simulink model "IEEE30_case"  (R2024b)
settings: Solver=FixedStepAuto  StartTime=0  StopTime=5  FixedStep=1e-7  RelTol=1e-3
values from neighbouring files (symbols this model uses):
  GFL_DFIG_7_C_bus = 0.08    [IEEE30_case_parameters.m]
  GFL_DFIG_7_D_mutual = 2.500000e+3    (= 2500)    [IEEE30_case_parameters.m]
  GFL_DFIG_7_f0 = 60    [IEEE30_case_parameters.m]
  GFL_DFIG_7_gPLLi = 3200    [IEEE30_case_parameters.m]
  GFL_DFIG_7_gPLLp = 650    [IEEE30_case_parameters.m]
  GFL_DFIG_7_H_WT = 0.4    [IEEE30_case_parameters.m]
  GFL_DFIG_7_Hg = 0.8    [IEEE30_case_parameters.m]
  GFL_DFIG_7_Igq_ref = 0    [IEEE30_case_parameters.m]
  GFL_DFIG_7_Ird_ref = 704.45696    [IEEE30_case_parameters.m]
  GFL_DFIG_7_KI_V = -300000    [IEEE30_case_parameters.m]
  GFL_DFIG_7_KP_V = -1000    [IEEE30_case_parameters.m]
  GFL_DFIG_7_Ksh = 1.254300e+4    (= 12543)    [IEEE30_case_parameters.m]
  GFL_DFIG_7_Lg = 0.000483    [IEEE30_case_parameters.m]
  GFL_DFIG_7_Lm_pu = 4    [IEEE30_case_parameters.m]
  GFL_DFIG_7_N = 100    [IEEE30_case_parameters.m]
  GFL_DFIG_7_p = 2    [IEEE30_case_parameters.m]
  GFL_DFIG_7_Pitch = 0    [IEEE30_case_parameters.m]
  GFL_DFIG_7_R = 44    [IEEE30_case_parameters.m]
  GFL_DFIG_7_Rg = 2.000000e-5    (= 2e-05)    [IEEE30_case_parameters.m]
  GFL_DFIG_7_rho = 1.225    [IEEE30_case_parameters.m]
  GFL_DFIG_7_rPLLi = 4500    [IEEE30_case_parameters.m]
  GFL_DFIG_7_rPLLp = 620    [IEEE30_case_parameters.m]
  GFL_DFIG_7_Rs_pu = 0.011    [IEEE30_case_parameters.m]
  GFL_DFIG_7_Sbase = 2.000000e+6    (= 2000000)    [IEEE30_case_parameters.m]
  GFL_DFIG_7_ugq_ref = 0    [IEEE30_case_parameters.m]
  GFL_DFIG_7_usd_ref = 0    [IEEE30_case_parameters.m]
  GFL_DFIG_7_Vbase = 690    [IEEE30_case_parameters.m]
  GFL_DFIG_7_Vdc_ref = 1200    [IEEE30_case_parameters.m]
  GFL_DFIG_7_wind = 12    [IEEE30_case_parameters.m]
  GFL_DFIG_7_wm_ref = 518.184209    [IEEE30_case_parameters.m]
  SG_D_13_D = 0.01056    [IEEE30_case_parameters.m]
  SG_D_13_EnableSaturation = 0    [IEEE30_case_parameters.m]
  SG_D_13_f0 = 60    [IEEE30_case_parameters.m]
  SG_D_13_H = 7.5    [IEEE30_case_parameters.m]
  SG_D_13_K_A = 20    [IEEE30_case_parameters.m]
  SG_D_13_K_E = 1.000000e+1    (= 10)    [IEEE30_case_parameters.m]
  SG_D_13_K_F = 2.363    [IEEE30_case_parameters.m]
  SG_D_13_K_s = 0.5    [IEEE30_case_parameters.m]
  SG_D_13_R_a = 0.001088    [IEEE30_case_parameters.m]
  SG_D_13_S_A = 1    [IEEE30_case_parameters.m]
  SG_D_13_S_B = 0.103    [IEEE30_case_parameters.m]
  SG_D_13_S_N = 10.659857    [IEEE30_case_parameters.m]
  SG_D_13_SpeedPara = 200    [IEEE30_case_parameters.m]
  SG_D_13_T_0 = 0.370163    [IEEE30_case_parameters.m]
  SG_D_13_T_1 = 0.3    [IEEE30_case_parameters.m]
  SG_D_13_T_2 = 0.05    [IEEE30_case_parameters.m]
  SG_D_13_T_3 = 0.02    [IEEE30_case_parameters.m]
  SG_D_13_T_4 = 0.005    [IEEE30_case_parameters.m]
  SG_D_13_T_A = 0.02    [IEEE30_case_parameters.m]
  SG_D_13_T_dd = 8.000000e+0    (= 8)    [IEEE30_case_parameters.m]
  SG_D_13_T_ddd = 0.04    [IEEE30_case_parameters.m]
  SG_D_13_T_E = 0.314    [IEEE30_case_parameters.m]
  SG_D_13_T_F = 0.35    [IEEE30_case_parameters.m]
  SG_D_13_T_qd = 0.8    [IEEE30_case_parameters.m]
  SG_D_13_T_qdd = 0.02    [IEEE30_case_parameters.m]
  SG_D_13_T_speed = 0.1    [IEEE30_case_parameters.m]
  SG_D_13_T_w = 0.5    [IEEE30_case_parameters.m]
  SG_D_13_V_ref = 1.696619    [IEEE30_case_parameters.m]
  SG_D_13_w_ref = 376.991118    [IEEE30_case_parameters.m]
  SG_D_13_x_d = 1.9    [IEEE30_case_parameters.m]
  SG_D_13_x_dd = 0.302    [IEEE30_case_parameters.m]
  SG_D_13_x_ddd = 0.204    [IEEE30_case_parameters.m]
  SG_D_13_x_l = 0.05    [IEEE30_case_parameters.m]
  SG_D_13_x_q = 1.3    [IEEE30_case_parameters.m]
  SG_D_13_x_qd = 0.5    [IEEE30_case_parameters.m]
  SG_D_13_x_qdd = 0.3    [IEEE30_case_parameters.m]
  SG_D_1_D = 0.01056    [IEEE30_case_parameters.m]
  SG_D_1_EnableSaturation = 0    [IEEE30_case_parameters.m]
  SG_D_1_f0 = 60    [IEEE30_case_parameters.m]
  SG_D_1_H = 7.5    [IEEE30_case_parameters.m]
  SG_D_1_K_A = 20    [IEEE30_case_parameters.m]
  SG_D_1_K_E = 1.000000e+1    (= 10)    [IEEE30_case_parameters.m]
  SG_D_1_K_F = 2.363    [IEEE30_case_parameters.m]
  SG_D_1_K_s = 0.5    [IEEE30_case_parameters.m]
  SG_D_1_R_a = 0.001088    [IEEE30_case_parameters.m]
  SG_D_1_S_A = 1    [IEEE30_case_parameters.m]
  SG_D_1_S_B = 0.103    [IEEE30_case_parameters.m]
  SG_D_1_S_N = 10.659857    [IEEE30_case_parameters.m]
  SG_D_1_SpeedPara = 200    [IEEE30_case_parameters.m]
  SG_D_1_T_0 = 0.259812    [IEEE30_case_parameters.m]
  SG_D_1_T_1 = 0.3    [IEEE30_case_parameters.m]
  SG_D_1_T_2 = 0.05    [IEEE30_case_parameters.m]
  SG_D_1_T_3 = 0.02    [IEEE30_case_parameters.m]
  SG_D_1_T_4 = 0.005    [IEEE30_case_parameters.m]
  SG_D_1_T_A = 0.02    [IEEE30_case_parameters.m]
  SG_D_1_T_dd = 8.000000e+0    (= 8)    [IEEE30_case_parameters.m]
  SG_D_1_T_ddd = 0.04    [IEEE30_case_parameters.m]
  SG_D_1_T_E = 0.314    [IEEE30_case_parameters.m]
  SG_D_1_T_F = 0.35    [IEEE30_case_parameters.m]
  SG_D_1_T_qd = 0.8    [IEEE30_case_parameters.m]
  SG_D_1_T_qdd = 0.02    [IEEE30_case_parameters.m]
  SG_D_1_T_speed = 0.1    [IEEE30_case_parameters.m]
  SG_D_1_T_w = 0.5    [IEEE30_case_parameters.m]
  SG_D_1_V_ref = 1.544107    [IEEE30_case_parameters.m]
  SG_D_1_w_ref = 376.991118    [IEEE30_case_parameters.m]
  SG_D_1_x_d = 1.9    [IEEE30_case_parameters.m]
  SG_D_1_x_dd = 0.302    [IEEE30_case_parameters.m]
  SG_D_1_x_ddd = 0.204    [IEEE30_case_parameters.m]
  SG_D_1_x_l = 0.05    [IEEE30_case_parameters.m]
  SG_D_1_x_q = 1.3    [IEEE30_case_parameters.m]
  SG_D_1_x_qd = 0.5    [IEEE30_case_parameters.m]
  SG_D_1_x_qdd = 0.3    [IEEE30_case_parameters.m]
  SG_D_22_D = 0.01056    [IEEE30_case_parameters.m]
  SG_D_22_EnableSaturation = 0    [IEEE30_case_parameters.m]
  SG_D_22_f0 = 60    [IEEE30_case_parameters.m]
  SG_D_22_H = 7.5    [IEEE30_case_parameters.m]
  SG_D_22_K_A = 20    [IEEE30_case_parameters.m]
  SG_D_22_K_E = 1.000000e+1    (= 10)    [IEEE30_case_parameters.m]
  SG_D_22_K_F = 2.363    [IEEE30_case_parameters.m]
  SG_D_22_K_s = 0.5    [IEEE30_case_parameters.m]
  SG_D_22_R_a = 0.001088    [IEEE30_case_parameters.m]
  SG_D_22_S_A = 1    [IEEE30_case_parameters.m]
  SG_D_22_S_B = 0.103    [IEEE30_case_parameters.m]
  SG_D_22_S_N = 10.659857    [IEEE30_case_parameters.m]
  SG_D_22_SpeedPara = 200    [IEEE30_case_parameters.m]
  SG_D_22_T_0 = 0.216121    [IEEE30_case_parameters.m]
  SG_D_22_T_1 = 0.3    [IEEE30_case_parameters.m]
  SG_D_22_T_2 = 0.05    [IEEE30_case_parameters.m]
  SG_D_22_T_3 = 0.02    [IEEE30_case_parameters.m]
  SG_D_22_T_4 = 0.005    [IEEE30_case_parameters.m]
  ... (+126 more)
(part 23 of 27)

== system IEEE30_case/SG_D_22/d_w_SG_D_22_block ==
  note: d_w_SG_D_22 in IEEE30_case
      | $\frac{2\,\pi \,T_{m,\mathrm{SG},D,22}\,f_{0}-D\,\left(w_{\mathrm{SG},D,22}-2\,\pi \,f_{0}\right)+2\,\pi \,f_{0}\,\left(\frac{\psi _{d,\mathrm{SG},D,22}\,\left(\psi _{q,\mathrm{SG},D,22}+\frac{\psi _{\mathrm{gq},\mathrm{SG},D,22}\,\left(x_{l}-x_{\mathrm{qdd}}\right)}{x_{l}-x_{\mathrm{qd}}}+\frac{\psi _{\mathrm{kq},\mathrm{SG},D,22}\,\left(x_{\mathrm{qd}}-x_{\mathrm{qdd}}\right)}{x_{l}-x_{\mathrm{qd}}}\right)}{x_{\mathrm{qdd}}}+\frac{\psi _{q,\mathrm{SG},D,22}\,\left(\frac{\psi _{\mathrm{1d},\mathrm{SG},D,22}\,\left(x_{\mathrm{dd}}-x_{\mathrm{ddd}}\right)}{x_{\mathrm{dd}}-x_{l}}-\psi _{d,\mathrm{SG},D,22}+\frac{\psi _{\mathrm{fd},\mathrm{SG},D,22}\,\left(x_{\mathrm{ddd}}-x_{l}\right)}{x_{\mathrm{dd}}-x_{l}}\right)}{x_{\mathrm{ddd}}}\right)}{2\,H}$
      | Automatically generated on 2025-11-01 18:36:16 .
  State_w_SG_D_22_fa999 : Inport
  State_T_m_SG_D_22_7e244 : Inport  Port=2
  State_psi_d_SG_D_22_73560 : Inport  Port=3
  State_psi_gq_SG_D_22_bb4d3 : Inport  Port=4
  State_psi_kq_SG_D_22_23ee7 : Inport  Port=5
  State_psi_q_SG_D_22_4ef4a : Inport  Port=6
  State_psi_q_SG_D_22_8c90d : Inport  Port=7
  State_psi_1d_SG_D_22_62d4d : Inport  Port=8
  State_psi_d_SG_D_22_0b647 : Inport  Port=9
  State_psi_fd_SG_D_22_b8daa : Inport  Port=10
  Add_01781 : Sum
  Add_114db : Sum
  Add_20ea4 : Sum
  Add_483be : Sum
  Add_4e463 : Sum
  Add_6d455 : Sum
  Add_81a44 : Sum
  Add_86346 : Sum
  Constant_-1_0835d : Constant  Value=-1
  Constant_-1_479f7 : Constant  Value=-1
  Constant_-1_4ac95 : Constant  Value=-1
  Constant_-1_7f41a : Constant  Value=-1
  Constant_-1_aceb8 : Constant  Value=-1
  Constant_-1_ccaa9 : Constant  Value=-1
  Constant_-2.0_91187 : Constant  Value=-2.0
  Constant_2.0_035fa : Constant  Value=2.0
  Constant_2.0_a509c : Constant  Value=2.0
  Constant_2.0_ee757 : Constant  Value=2.0
  Constant_D_fe311 : Constant  Value=D
  Constant_H_e5a3f : Constant  Value=H
  Constant_f0_a860d : Constant  Value=f0
  Constant_f0_ea105 : Constant  Value=f0
  Constant_f0_f8cec : Constant  Value=f0
  Constant_pi_04ed5 : Constant  Value=pi
  Constant_pi_3b5ba : Constant  Value=pi
  Constant_pi_ac5d2 : Constant  Value=pi
  Constant_x_dd_18a9f : Constant  Value=x_dd
  Constant_x_dd_2d7c4 : Constant  Value=x_dd
  Constant_x_dd_f986c : Constant  Value=x_dd
  Constant_x_ddd_45241 : Constant  Value=x_ddd
  Constant_x_ddd_a28f3 : Constant  Value=x_ddd
  Constant_x_ddd_a3165 : Constant  Value=x_ddd
  Constant_x_l_63a6c : Constant  Value=x_l
  Constant_x_l_bdb3a : Constant  Value=x_l
  Constant_x_l_cf755 : Constant  Value=x_l
  Constant_x_l_f1425 : Constant  Value=x_l
  Constant_x_l_f1fd2 : Constant  Value=x_l
  Constant_x_l_fc6ff : Constant  Value=x_l
  Constant_x_qd_268f7 : Constant  Value=x_qd
  Constant_x_qd_da002 : Constant  Value=x_qd
  Constant_x_qd_f1c3d : Constant  Value=x_qd
  Constant_x_qdd_3f849 : Constant  Value=x_qdd
  Constant_x_qdd_6cd35 : Constant  Value=x_qdd
  Constant_x_qdd_be498 : Constant  Value=x_qdd
  Divide_3b27e : Product  Inputs=*/
  Divide_430ae : Product  Inputs=*/
  Divide_4d63e : Product  Inputs=*/
  Divide_52483 : Product  Inputs=*/
  Divide_81c96 : Product  Inputs=*/
  Divide_e8000 : Product  Inputs=*/
  Divide_f9364 : Product  Inputs=*/
  Product_01bdb : Product
  Product_02883 : Product
  Product_1403b : Product
  Product_18bc2 : Product
  Product_21e43 : Product
  Product_2d9f5 : Product
  Product_2ff7e : Product
  Product_38649 : Product
  Product_4a0cf : Product
  Product_5b6d3 : Product
  Product_5c5b0 : Product
  Product_65d33 : Product
  Product_8f3f9 : Product
  Product_957ce : Product
  Product_9a778 : Product
  Product_a81af : Product
  Product_a8898 : Product
  Product_ac4c6 : Product
  Product_bec86 : Product
  Product_c664f : Product
  Product_fe5c2 : Product
  Product_ff451 : Product
  Subtract_04f57 : Sum  Inputs=+-
  Subtract_20ea5 : Sum  Inputs=+-
  Subtract_288bf : Sum  Inputs=+-
  Subtract_3d095 : Sum  Inputs=+-
  Subtract_567d8 : Sum  Inputs=+-
  Subtract_7ec3e : Sum  Inputs=+-
  Subtract_f02a9 : Sum  Inputs=+-
  Subtract_f0d31 : Sum  Inputs=+-
  Blockout_d_w_SG_D_22_fc61f : Outport
  wires:
  Product_1403b/1 -> Product_65d33/1
  Constant_x_qdd_6cd35/1 -> Add_86346/2
  Constant_-1_0835d/1 -> Product_01bdb/1
  Product_01bdb/1 -> Add_86346/1
  Constant_x_l_cf755/1 -> Product_01bdb/2
  Product_2ff7e/1 -> Add_01781/1
  State_psi_q_SG_D_22_4ef4a/1 -> Add_20ea4/2
  Constant_-1_7f41a/1 -> Product_5b6d3/1
  State_psi_1d_SG_D_22_62d4d/1 -> Product_bec86/2
  Constant_x_qd_f1c3d/1 -> Subtract_7ec3e/1
  Constant_x_l_63a6c/1 -> Product_5b6d3/2
  Constant_x_qdd_be498/1 -> Subtract_7ec3e/2
  Divide_e8000/1 -> Add_114db/1
  Constant_-1_479f7/1 -> Product_ff451/1
  Constant_x_l_bdb3a/1 -> Product_ff451/2
  Constant_-1_ccaa9/1 -> Product_bec86/1
  Constant_x_dd_f986c/1 -> Subtract_04f57/1
  Product_ff451/1 -> Add_483be/1
  Constant_x_ddd_a3165/1 -> Subtract_04f57/2
  State_psi_gq_SG_D_22_bb4d3/1 -> Product_18bc2/1
  Constant_x_l_f1fd2/1 -> Subtract_567d8/2
  Add_86346/1 -> Product_18bc2/2
  Constant_-2.0_91187/1 -> Product_9a778/1
  Product_5b6d3/1 -> Add_81a44/1
  Constant_x_qd_268f7/1 -> Add_81a44/2
  Subtract_f0d31/1 -> Product_2d9f5/2
  State_psi_kq_SG_D_22_23ee7/1 -> Product_4a0cf/1
  Subtract_7ec3e/1 -> Product_4a0cf/2
  Constant_x_qd_da002/1 -> Add_483be/2
  Subtract_04f57/1 -> Product_a81af/2
  Product_bec86/1 -> Product_a81af/1
  Constant_x_dd_2d7c4/1 -> Subtract_f02a9/1
  State_w_SG_D_22_fa999/1 -> Add_01781/2
  Product_02883/1 -> Product_fe5c2/1
  Constant_x_l_f1425/1 -> Subtract_f02a9/2
  Constant_x_ddd_a28f3/1 -> Subtract_567d8/1
  Product_18bc2/1 -> Divide_52483/1
  Add_81a44/1 -> Divide_52483/2
  Product_4a0cf/1 -> Divide_f9364/1
  Add_483be/1 -> Divide_f9364/2
  Product_a81af/1 -> Divide_e8000/1
  Add_01781/1 -> Product_65d33/2
  Subtract_f02a9/1 -> Divide_e8000/2
  Constant_2.0_a509c/1 -> Product_38649/1
  State_psi_fd_SG_D_22_b8daa/1 -> Product_c664f/1
  State_psi_d_SG_D_22_73560/1 -> Product_02883/2
  Subtract_567d8/1 -> Product_c664f/2
  Constant_x_dd_18a9f/1 -> Subtract_20ea5/1
  Constant_x_l_fc6ff/1 -> Subtract_20ea5/2
  Divide_52483/1 -> Subtract_3d095/1
  Divide_f9364/1 -> Subtract_3d095/2
  Constant_D_fe311/1 -> Product_1403b/2
  State_psi_d_SG_D_22_0b647/1 -> Add_114db/2
  Product_c664f/1 -> Divide_430ae/1
  Subtract_20ea5/1 -> Divide_430ae/2
  Constant_pi_3b5ba/1 -> Product_9a778/2
  Constant_-1_4ac95/1 -> Product_02883/1
  Subtract_3d095/1 -> Add_20ea4/1
  Add_114db/1 -> Subtract_f0d31/1
  Divide_430ae/1 -> Subtract_f0d31/2
  Constant_-1_aceb8/1 -> Product_1403b/1
  Product_9a778/1 -> Product_2ff7e/1
  Constant_f0_f8cec/1 -> Product_2ff7e/2
  Constant_pi_ac5d2/1 -> Product_38649/2
  Add_20ea4/1 -> Product_fe5c2/2
  State_psi_q_SG_D_22_8c90d/1 -> Product_2d9f5/1
  Product_38649/1 -> Product_5c5b0/1
  State_T_m_SG_D_22_7e244/1 -> Product_5c5b0/2
  Constant_2.0_035fa/1 -> Product_ac4c6/1
  Constant_pi_04ed5/1 -> Product_ac4c6/2
  Product_fe5c2/1 -> Divide_3b27e/1
  Constant_x_qdd_3f849/1 -> Divide_3b27e/2
  Product_2d9f5/1 -> Divide_81c96/1
  Constant_x_ddd_45241/1 -> Divide_81c96/2
  Product_5c5b0/1 -> Product_21e43/1
  Constant_f0_a860d/1 -> Product_21e43/2
  Product_ac4c6/1 -> Product_a8898/1
  Constant_f0_ea105/1 -> Product_a8898/2
  Subtract_288bf/1 -> Divide_4d63e/1
  Divide_3b27e/1 -> Add_4e463/1
  Divide_81c96/1 -> Add_4e463/2
  Product_65d33/1 -> Add_6d455/1
  Product_21e43/1 -> Add_6d455/2
  Product_a8898/1 -> Product_8f3f9/1
  Product_957ce/1 -> Divide_4d63e/2
  Add_4e463/1 -> Product_8f3f9/2
  Add_6d455/1 -> Subtract_288bf/1
  Product_8f3f9/1 -> Subtract_288bf/2
  Constant_2.0_ee757/1 -> Product_957ce/1
  Constant_H_e5a3f/1 -> Product_957ce/2
  Divide_4d63e/1 -> Blockout_d_w_SG_D_22_fc61f/1

== system IEEE30_case/SG_D_22/i_d_SG_D_22_block ==
  note: i_d_SG_D_22 in IEEE30_case
      | $\frac{\sin\left(\theta _{\mathrm{SG},D,22}\right)\,\left(\frac{\psi _{\mathrm{1d},\mathrm{SG},D,22}\,\left(x_{\mathrm{dd}}-x_{\mathrm{ddd}}\right)}{x_{\mathrm{dd}}-x_{l}}-\psi _{d,\mathrm{SG},D,22}+\frac{\psi _{\mathrm{fd},\mathrm{SG},D,22}\,\left(x_{\mathrm{ddd}}-x_{l}\right)}{x_{\mathrm{dd}}-x_{l}}\right)}{x_{\mathrm{ddd}}}-\frac{\cos\left(\theta _{\mathrm{SG},D,22}\right)\,\left(\psi _{q,\mathrm{SG},D,22}+\frac{\psi _{\mathrm{gq},\mathrm{SG},D,22}\,\left(x_{l}-x_{\mathrm{qdd}}\right)}{x_{l}-x_{\mathrm{qd}}}+\frac{\psi _{\mathrm{kq},\mathrm{SG},D,22}\,\left(x_{\mathrm{qd}}-x_{\mathrm{qdd}}\right)}{x_{l}-x_{\mathrm{qd}}}\right)}{x_{\mathrm{qdd}}}$
      | Automatically generated on 2025-11-01 18:36:38 .
  State_psi_gq_SG_D_22_058cc : Inport
  State_psi_kq_SG_D_22_d07e7 : Inport  Port=2
  State_psi_q_SG_D_22_9e84b : Inport  Port=3
  State_theta_SG_D_22_792f8 : Inport  Port=4
  State_psi_1d_SG_D_22_424d2 : Inport  Port=5
  State_psi_d_SG_D_22_8fd04 : Inport  Port=6
  State_psi_fd_SG_D_22_0bdd4 : Inport  Port=7
  State_theta_SG_D_22_e389e : Inport  Port=8
  Add_17bb1 : Sum
  Add_9e138 : Sum
  Add_9ec15 : Sum
  Add_a4406 : Sum
  Add_fa013 : Sum
  Constant_-1_1b914 : Constant  Value=-1
  Constant_-1_1c5f4 : Constant  Value=-1
  Constant_-1_9c796 : Constant  Value=-1
  Constant_-1_be524 : Constant  Value=-1
  Constant_-1_c767e : Constant  Value=-1
  Constant_x_dd_2ada7 : Constant  Value=x_dd
  Constant_x_dd_6ce68 : Constant  Value=x_dd
  Constant_x_dd_f2494 : Constant  Value=x_dd
  Constant_x_ddd_b379c : Constant  Value=x_ddd
  Constant_x_ddd_e6ff5 : Constant  Value=x_ddd
  Constant_x_ddd_f5fa1 : Constant  Value=x_ddd
  Constant_x_l_2eb3d : Constant  Value=x_l
  Constant_x_l_4962d : Constant  Value=x_l
  Constant_x_l_522f3 : Constant  Value=x_l
  Constant_x_l_5c091 : Constant  Value=x_l
  Constant_x_l_abada : Constant  Value=x_l
  Constant_x_l_ce708 : Constant  Value=x_l
  Constant_x_qd_39f13 : Constant  Value=x_qd
  Constant_x_qd_4e741 : Constant  Value=x_qd
  Constant_x_qd_f4057 : Constant  Value=x_qd
  Constant_x_qdd_1c041 : Constant  Value=x_qdd
  Constant_x_qdd_2d68a : Constant  Value=x_qdd
  Constant_x_qdd_e4405 : Constant  Value=x_qdd
  Divide_3d9a7 : Product  Inputs=*/
  Divide_9696c : Product  Inputs=*/
  Divide_9f5e7 : Product  Inputs=*/
  Divide_bfb6c : Product  Inputs=*/
  Divide_cac9e : Product  Inputs=*/
  Divide_eb2c3 : Product  Inputs=*/
  MathFunc_cos_35b8d : Trigonometry  Operator=cos
  MathFunc_sin_08b67 : Trigonometry
  Product_01cb8 : Product
  Product_44b7e : Product
  Product_4ded6 : Product
  Product_55153 : Product
  Product_79e31 : Product
  Product_8bd60 : Product
  Product_ac25e : Product
  Product_cbc80 : Product
  Product_eaafb : Product
  Product_f1ef4 : Product
  Product_fc02d : Product
  Subtract_0887a : Sum  Inputs=+-
  Subtract_25a61 : Sum  Inputs=+-
  Subtract_59e0e : Sum  Inputs=+-
  Subtract_851e2 : Sum  Inputs=+-
  Subtract_86be8 : Sum  Inputs=+-
  Subtract_a7935 : Sum  Inputs=+-
  Subtract_a8970 : Sum  Inputs=+-
  Subtract_b239c : Sum  Inputs=+-
  Blockout_i_d_SG_D_22_9977f : Outport
  wires:
  Product_f1ef4/1 -> Divide_bfb6c/1
  Constant_-1_be524/1 -> Product_44b7e/1
  Constant_-1_c767e/1 -> Product_79e31/1
  Constant_x_l_2eb3d/1 -> Product_44b7e/2
  Constant_x_dd_6ce68/1 -> Subtract_86be8/1
  Product_ac25e/1 -> Add_9e138/1
  Constant_x_qdd_e4405/1 -> Add_9ec15/2
  Product_44b7e/1 -> Add_9ec15/1
  Constant_-1_9c796/1 -> Product_cbc80/1
  Subtract_0887a/1 -> Product_01cb8/2
  Constant_x_l_ce708/1 -> Product_cbc80/2
  MathFunc_sin_08b67/1 -> Product_8bd60/2
  Constant_x_qd_4e741/1 -> Add_fa013/2
  Constant_x_qd_f4057/1 -> Subtract_0887a/1
  Subtract_25a61/1 -> Product_4ded6/2
  Constant_x_qdd_2d68a/1 -> Subtract_0887a/2
  Constant_-1_1c5f4/1 -> Product_ac25e/1
  Constant_x_dd_2ada7/1 -> Subtract_a8970/1
  Constant_x_l_4962d/1 -> Product_ac25e/2
  Add_9e138/1 -> Divide_9696c/2
  State_psi_gq_SG_D_22_058cc/1 -> Product_fc02d/1
  Add_9ec15/1 -> Product_fc02d/2
  Product_4ded6/1 -> Divide_eb2c3/1
  State_psi_1d_SG_D_22_424d2/1 -> Product_79e31/2
  Product_cbc80/1 -> Add_fa013/1
  State_psi_kq_SG_D_22_d07e7/1 -> Product_01cb8/1
  Constant_x_qd_39f13/1 -> Add_9e138/2
  Divide_9f5e7/1 -> Subtract_59e0e/2
  Constant_x_ddd_b379c/1 -> Subtract_86be8/2
  Product_fc02d/1 -> Divide_cac9e/1
  Product_79e31/1 -> Product_f1ef4/1
  Add_fa013/1 -> Divide_cac9e/2
  Constant_x_ddd_f5fa1/1 -> Subtract_25a61/1
  Product_01cb8/1 -> Divide_9696c/1
  Constant_x_qdd_1c041/1 -> Divide_3d9a7/2
  Subtract_86be8/1 -> Product_f1ef4/2
  State_psi_q_SG_D_22_9e84b/1 -> Add_a4406/2
  Divide_9696c/1 -> Subtract_851e2/2
  Constant_x_dd_f2494/1 -> Subtract_a7935/1
  Constant_x_l_5c091/1 -> Subtract_a7935/2
  Add_17bb1/1 -> Subtract_b239c/1
  Constant_x_l_522f3/1 -> Subtract_25a61/2
  Divide_cac9e/1 -> Subtract_851e2/1
  Subtract_a7935/1 -> Divide_bfb6c/2
  State_psi_fd_SG_D_22_0bdd4/1 -> Product_4ded6/1
  Subtract_b239c/1 -> Product_8bd60/1
  Constant_x_l_abada/1 -> Subtract_a8970/2
  Subtract_851e2/1 -> Add_a4406/1
  Divide_bfb6c/1 -> Add_17bb1/1
  State_psi_d_SG_D_22_8fd04/1 -> Add_17bb1/2
  Product_55153/1 -> Divide_3d9a7/1
  Subtract_a8970/1 -> Divide_eb2c3/2
  Constant_-1_1b914/1 -> Product_eaafb/1
  Add_a4406/1 -> Product_eaafb/2
  MathFunc_cos_35b8d/1 -> Product_55153/2
  State_theta_SG_D_22_792f8/1 -> MathFunc_cos_35b8d/1
  Divide_eb2c3/1 -> Subtract_b239c/2
  State_theta_SG_D_22_e389e/1 -> MathFunc_sin_08b67/1
  Subtract_59e0e/1 -> Blockout_i_d_SG_D_22_9977f/1
  Product_eaafb/1 -> Product_55153/1
  Product_8bd60/1 -> Divide_9f5e7/1
  Constant_x_ddd_e6ff5/1 -> Divide_9f5e7/2
  Divide_3d9a7/1 -> Subtract_59e0e/1

== system IEEE30_case/SG_D_22/i_q_SG_D_22_block ==
  note: i_q_SG_D_22 in IEEE30_case
      | $-\frac{\sin\left(\theta _{\mathrm{SG},D,22}\right)\,\left(\psi _{q,\mathrm{SG},D,22}+\frac{\psi _{\mathrm{gq},\mathrm{SG},D,22}\,\left(x_{l}-x_{\mathrm{qdd}}\right)}{x_{l}-x_{\mathrm{qd}}}+\frac{\psi _{\mathrm{kq},\mathrm{SG},D,22}\,\left(x_{\mathrm{qd}}-x_{\mathrm{qdd}}\right)}{x_{l}-x_{\mathrm{qd}}}\right)}{x_{\mathrm{qdd}}}-\frac{\cos\left(\theta _{\mathrm{SG},D,22}\right)\,\left(\frac{\psi _{\mathrm{1d},\mathrm{SG},D,22}\,\left(x_{\mathrm{dd}}-x_{\mathrm{ddd}}\right)}{x_{\mathrm{dd}}-x_{l}}-\psi _{d,\mathrm{SG},D,22}+\frac{\psi _{\mathrm{fd},\mathrm{SG},D,22}\,\left(x_{\mathrm{ddd}}-x_{l}\right)}{x_{\mathrm{dd}}-x_{l}}\right)}{x_{\mathrm{ddd}}}$
      | Automatically generated on 2025-11-01 18:36:42 .
  State_psi_gq_SG_D_22_6529e : Inport
  State_psi_kq_SG_D_22_c8bb0 : Inport  Port=2
  State_psi_q_SG_D_22_a1550 : Inport  Port=3
  State_theta_SG_D_22_35a4e : Inport  Port=4
  State_psi_1d_SG_D_22_666cb : Inport  Port=5
  State_psi_d_SG_D_22_f015b : Inport  Port=6
  State_psi_fd_SG_D_22_6d852 : Inport  Port=7
  State_theta_SG_D_22_5c4fb : Inport  Port=8
  Add_091c4 : Sum
  Add_0b43f : Sum
  Add_0b988 : Sum
  Add_7646a : Sum
  Add_975f9 : Sum
  Add_de373 : Sum
  Constant_-1_328d6 : Constant  Value=-1
  Constant_-1_6e275 : Constant  Value=-1
  Constant_-1_8b2f0 : Constant  Value=-1
  Constant_-1_c5b86 : Constant  Value=-1
  Constant_-1_edc7d : Constant  Value=-1
  Constant_x_dd_216a6 : Constant  Value=x_dd
  Constant_x_dd_8efda : Constant  Value=x_dd
  Constant_x_dd_ced0e : Constant  Value=x_dd
  Constant_x_ddd_6ea92 : Constant  Value=x_ddd
  Constant_x_ddd_7893e : Constant  Value=x_ddd
  Constant_x_ddd_c710b : Constant  Value=x_ddd
  Constant_x_l_0cede : Constant  Value=x_l
  Constant_x_l_43b7c : Constant  Value=x_l
  Constant_x_l_803c9 : Constant  Value=x_l
  Constant_x_l_bd6c4 : Constant  Value=x_l
  Constant_x_l_d96a4 : Constant  Value=x_l
  Constant_x_l_e3511 : Constant  Value=x_l
  Constant_x_qd_0fd2b : Constant  Value=x_qd
  Constant_x_qd_4274d : Constant  Value=x_qd
  Constant_x_qd_d3432 : Constant  Value=x_qd
  Constant_x_qdd_0101f : Constant  Value=x_qdd
  Constant_x_qdd_5f2dd : Constant  Value=x_qdd
  Constant_x_qdd_afa35 : Constant  Value=x_qdd
  Divide_27393 : Product  Inputs=*/
  Divide_396b9 : Product  Inputs=*/
  Divide_5d266 : Product  Inputs=*/
  Divide_6668b : Product  Inputs=*/
  Divide_b6289 : Product  Inputs=*/
  Divide_fc06a : Product  Inputs=*/
  MathFunc_cos_8f398 : Trigonometry  Operator=cos
  MathFunc_sin_55e9c : Trigonometry
  Product_179a3 : Product
  Product_2952f : Product
  Product_36126 : Product
  Product_38281 : Product
  Product_38531 : Product
  Product_52de5 : Product
  Product_5b153 : Product
  Product_90a31 : Product
  Product_a5766 : Product
  Product_d1944 : Product
  Product_df09f : Product
  Subtract_2bb11 : Sum  Inputs=+-
  Subtract_46af6 : Sum  Inputs=+-
  Subtract_5be83 : Sum  Inputs=+-
  Subtract_7b3a3 : Sum  Inputs=+-
  Subtract_823cd : Sum  Inputs=+-
  Subtract_abeed : Sum  Inputs=+-
  Subtract_b356d : Sum  Inputs=+-
  Blockout_i_q_SG_D_22_b8c62 : Outport
  wires:
  Product_d1944/1 -> Divide_6668b/1
  Constant_x_l_d96a4/1 -> Product_5b153/2
  Product_179a3/1 -> Divide_27393/1
  Constant_-1_8b2f0/1 -> Product_5b153/1
  Product_df09f/1 -> Product_36126/1
  Product_5b153/1 -> Add_0b43f/1
  Constant_x_qdd_5f2dd/1 -> Subtract_7b3a3/2
  Constant_x_qdd_0101f/1 -> Add_0b43f/2
  Constant_-1_edc7d/1 -> Product_a5766/1
  Constant_x_l_bd6c4/1 -> Product_a5766/2
  Constant_x_qd_d3432/1 -> Subtract_7b3a3/1
  Constant_x_l_e3511/1 -> Subtract_b356d/2
  Constant_-1_6e275/1 -> Product_38531/1
  Constant_x_l_0cede/1 -> Product_38531/2
  State_psi_1d_SG_D_22_666cb/1 -> Product_df09f/2
  State_psi_gq_SG_D_22_6529e/1 -> Product_90a31/1
  Divide_5d266/1 -> Add_de373/1
  Add_0b43f/1 -> Product_90a31/2
  Add_de373/1 -> Blockout_i_q_SG_D_22_b8c62/1
  Product_a5766/1 -> Add_0b988/1
  Constant_x_qd_4274d/1 -> Add_0b988/2
  State_psi_kq_SG_D_22_c8bb0/1 -> Product_d1944/1
  Subtract_7b3a3/1 -> Product_d1944/2
  Product_38531/1 -> Add_091c4/1
  Subtract_b356d/1 -> Divide_396b9/2
  Constant_x_qd_0fd2b/1 -> Add_091c4/2
  Add_0b988/1 -> Divide_b6289/2
  Constant_-1_328d6/1 -> Product_df09f/1
  Constant_x_dd_216a6/1 -> Subtract_823cd/1
  Constant_x_ddd_7893e/1 -> Subtract_823cd/2
  Product_90a31/1 -> Divide_b6289/1
  Add_091c4/1 -> Divide_6668b/2
  State_psi_q_SG_D_22_a1550/1 -> Add_7646a/2
  Subtract_823cd/1 -> Product_36126/2
  Constant_x_dd_ced0e/1 -> Subtract_b356d/1
  Subtract_46af6/1 -> Product_2952f/2
  Constant_x_ddd_6ea92/1 -> Subtract_46af6/1
  Constant_x_l_43b7c/1 -> Subtract_46af6/2
  Divide_b6289/1 -> Subtract_abeed/1
  Divide_6668b/1 -> Subtract_abeed/2
  State_psi_d_SG_D_22_f015b/1 -> Add_975f9/2
  Product_36126/1 -> Divide_396b9/1
  Product_2952f/1 -> Divide_fc06a/1
  State_psi_fd_SG_D_22_6d852/1 -> Product_2952f/1
  Subtract_2bb11/1 -> Divide_fc06a/2
  Constant_x_dd_8efda/1 -> Subtract_2bb11/1
  Constant_x_l_803c9/1 -> Subtract_2bb11/2
  Subtract_abeed/1 -> Add_7646a/1
  Product_52de5/1 -> Product_38281/1
  Divide_396b9/1 -> Add_975f9/1
  Constant_-1_c5b86/1 -> Product_52de5/1
  Add_7646a/1 -> Product_52de5/2
  MathFunc_sin_55e9c/1 -> Product_38281/2
  State_theta_SG_D_22_35a4e/1 -> MathFunc_sin_55e9c/1
  Add_975f9/1 -> Subtract_5be83/1
  Divide_fc06a/1 -> Subtract_5be83/2
  MathFunc_cos_8f398/1 -> Product_179a3/2
  State_theta_SG_D_22_5c4fb/1 -> MathFunc_cos_8f398/1
  Subtract_5be83/1 -> Product_179a3/1
  Product_38281/1 -> Divide_5d266/1
  Constant_x_qdd_afa35/1 -> Divide_5d266/2
  Constant_x_ddd_c710b/1 -> Divide_27393/2
  Divide_27393/1 -> Add_de373/2

== system IEEE30_case/SG_D_22/theta_SG_D_22_out_block ==
  note: theta_SG_D_22_out in IEEE30_case
      | $\theta _{\mathrm{SG},D,22}$
      | Automatically generated on 2025-11-01 18:36:48 .
  State_theta_SG_D_22_89d34 : Inport
  Blockout_theta_SG_D_22_out_cf0c5 : Outport
  wires:
  State_theta_SG_D_22_89d34/1 -> Blockout_theta_SG_D_22_out_cf0c5/1

== system IEEE30_case/SG_D_22/w_SG_D_22_out_block ==
  note: w_SG_D_22_out in IEEE30_case
      | $w_{\mathrm{SG},D,22}$
      | Automatically generated on 2025-11-01 18:36:47 .
  State_w_SG_D_22_6ca8a : Inport
  Blockout_w_SG_D_22_out_8ba47 : Outport
  wires:
  State_w_SG_D_22_6ca8a/1 -> Blockout_w_SG_D_22_out_8ba47/1

== system IEEE30_case/SG_D_23/T_e_SG_D_23_block ==
  note: T_e_SG_D_23 in IEEE30_case
      | $-\frac{\psi _{d,\mathrm{SG},D,23}\,\left(\psi _{q,\mathrm{SG},D,23}+\frac{\psi _{\mathrm{gq},\mathrm{SG},D,23}\,\left(x_{l}-x_{\mathrm{qdd}}\right)}{x_{l}-x_{\mathrm{qd}}}+\frac{\psi _{\mathrm{kq},\mathrm{SG},D,23}\,\left(x_{\mathrm{qd}}-x_{\mathrm{qdd}}\right)}{x_{l}-x_{\mathrm{qd}}}\right)}{x_{\mathrm{qdd}}}-\frac{\psi _{q,\mathrm{SG},D,23}\,\left(\frac{\psi _{\mathrm{1d},\mathrm{SG},D,23}\,\left(x_{\mathrm{dd}}-x_{\mathrm{ddd}}\right)}{x_{\mathrm{dd}}-x_{l}}-\psi _{d,\mathrm{SG},D,23}+\frac{\psi _{\mathrm{fd},\mathrm{SG},D,23}\,\left(x_{\mathrm{ddd}}-x_{l}\right)}{x_{\mathrm{dd}}-x_{l}}\right)}{x_{\mathrm{ddd}}}$
      | Automatically generated on 2025-11-01 18:37:54 .
  State_psi_d_SG_D_23_826a4 : Inport
  State_psi_gq_SG_D_23_12628 : Inport  Port=2
  State_psi_kq_SG_D_23_f7b1e : Inport  Port=3
  State_psi_q_SG_D_23_c6c28 : Inport  Port=4
  State_psi_q_SG_D_23_65500 : Inport  Port=5
  State_psi_1d_SG_D_23_5b6b0 : Inport  Port=6
  State_psi_d_SG_D_23_8cfae : Inport  Port=7
  State_psi_fd_SG_D_23_2df9d : Inport  Port=8
  Add_17c51 : Sum
  Add_4c836 : Sum
  Add_64270 : Sum
  Add_7e1c0 : Sum
  Add_d65be : Sum
  Add_f6515 : Sum
  Constant_-1_3463a : Constant  Value=-1
  Constant_-1_56fd3 : Constant  Value=-1
  Constant_-1_755c0 : Constant  Value=-1
  Constant_-1_8e5c5 : Constant  Value=-1
  Constant_-1_a6549 : Constant  Value=-1
  Constant_x_dd_4a83c : Constant  Value=x_dd
  Constant_x_dd_90e1c : Constant  Value=x_dd
  Constant_x_dd_fedb0 : Constant  Value=x_dd
  Constant_x_ddd_9c197 : Constant  Value=x_ddd
  Constant_x_ddd_a3c28 : Constant  Value=x_ddd
  Constant_x_ddd_dddcf : Constant  Value=x_ddd
  Constant_x_l_95ca8 : Constant  Value=x_l
  Constant_x_l_ce350 : Constant  Value=x_l
  Constant_x_l_e425f : Constant  Value=x_l
  Constant_x_l_ed5da : Constant  Value=x_l
  Constant_x_l_f4faf : Constant  Value=x_l
  Constant_x_l_f9720 : Constant  Value=x_l
  Constant_x_qd_002a1 : Constant  Value=x_qd
  Constant_x_qd_31d68 : Constant  Value=x_qd
  Constant_x_qd_3ee38 : Constant  Value=x_qd
  Constant_x_qdd_2d6cc : Constant  Value=x_qdd
  Constant_x_qdd_40487 : Constant  Value=x_qdd
  Constant_x_qdd_e2840 : Constant  Value=x_qdd
  Divide_0e8c6 : Product  Inputs=*/
  Divide_10d51 : Product  Inputs=*/
  Divide_4991f : Product  Inputs=*/
  Divide_4b770 : Product  Inputs=*/
  Divide_780f9 : Product  Inputs=*/
  Divide_87dd8 : Product  Inputs=*/
  Product_13071 : Product
  Product_32682 : Product
  Product_485dd : Product
  Product_4bacf : Product
  Product_4f42c : Product
  Product_83b09 : Product
  Product_88620 : Product
  Product_9c765 : Product
  Product_a8dc3 : Product
  Product_be3d6 : Product
  Product_eade7 : Product
  Subtract_1590b : Sum  Inputs=+-
  Subtract_25dd9 : Sum  Inputs=+-
  Subtract_3282f : Sum  Inputs=+-
  Subtract_84155 : Sum  Inputs=+-
  Subtract_88456 : Sum  Inputs=+-
  Subtract_b6772 : Sum  Inputs=+-
  Subtract_e4bf3 : Sum  Inputs=+-
  Blockout_T_e_SG_D_23_908bc : Outport
  wires:
  Product_88620/1 -> Divide_4b770/1
  State_psi_q_SG_D_23_65500/1 -> Product_88620/1
  Constant_-1_a6549/1 -> Product_a8dc3/1
  Constant_x_l_ce350/1 -> Subtract_1590b/2
  Constant_x_l_f4faf/1 -> Product_a8dc3/2
  Product_485dd/1 -> Divide_780f9/1
  Constant_x_qdd_40487/1 -> Add_4c836/2
  State_psi_1d_SG_D_23_5b6b0/1 -> Product_13071/2
  Constant_-1_755c0/1 -> Product_4f42c/1
  Product_a8dc3/1 -> Add_4c836/1
  Constant_-1_56fd3/1 -> Product_4bacf/1
  Product_83b09/1 -> Divide_87dd8/1
  State_psi_fd_SG_D_23_2df9d/1 -> Product_485dd/1
  Constant_x_l_95ca8/1 -> Product_4bacf/2
  Constant_x_qd_3ee38/1 -> Subtract_e4bf3/1
  Constant_x_qdd_2d6cc/1 -> Subtract_e4bf3/2
  Constant_x_l_e425f/1 -> Product_4f42c/2
  State_psi_q_SG_D_23_c6c28/1 -> Add_f6515/2
  Product_13071/1 -> Product_be3d6/1
  Constant_-1_3463a/1 -> Product_13071/1
  Subtract_3282f/1 -> Product_be3d6/2
  Constant_x_dd_4a83c/1 -> Subtract_3282f/1
  Product_4f42c/1 -> Add_d65be/1
  Constant_x_ddd_dddcf/1 -> Subtract_3282f/2
  Constant_x_ddd_9c197/1 -> Divide_4b770/2
  State_psi_gq_SG_D_23_12628/1 -> Product_32682/1
  State_psi_d_SG_D_23_826a4/1 -> Product_eade7/2
  Add_4c836/1 -> Product_32682/2
  Product_4bacf/1 -> Add_64270/1
  Constant_x_qdd_e2840/1 -> Divide_87dd8/2
  Subtract_1590b/1 -> Product_485dd/2
  Constant_x_qd_31d68/1 -> Add_64270/2
  State_psi_kq_SG_D_23_f7b1e/1 -> Product_9c765/1
  Subtract_e4bf3/1 -> Product_9c765/2
  Constant_x_qd_002a1/1 -> Add_d65be/2
  Subtract_25dd9/1 -> Divide_10d51/2
  Constant_x_dd_90e1c/1 -> Subtract_25dd9/1
  Add_17c51/1 -> Subtract_88456/1
  Constant_x_l_f9720/1 -> Subtract_25dd9/2
  Constant_x_ddd_a3c28/1 -> Subtract_1590b/1
  Product_32682/1 -> Divide_4991f/1
  Subtract_b6772/1 -> Divide_780f9/2
  Add_64270/1 -> Divide_4991f/2
  Product_9c765/1 -> Divide_0e8c6/1
  Add_7e1c0/1 -> Blockout_T_e_SG_D_23_908bc/1
  Add_d65be/1 -> Divide_0e8c6/2
  Product_be3d6/1 -> Divide_10d51/1
  Constant_x_dd_fedb0/1 -> Subtract_b6772/1
  Constant_x_l_ed5da/1 -> Subtract_b6772/2
  Divide_4991f/1 -> Subtract_84155/1
  Divide_0e8c6/1 -> Subtract_84155/2
  State_psi_d_SG_D_23_8cfae/1 -> Add_17c51/2
  Divide_10d51/1 -> Add_17c51/1
  Constant_-1_8e5c5/1 -> Product_eade7/1
  Subtract_84155/1 -> Add_f6515/1
  Divide_780f9/1 -> Subtract_88456/2
  Product_eade7/1 -> Product_83b09/1
  Add_f6515/1 -> Product_83b09/2
  Divide_87dd8/1 -> Add_7e1c0/1
  Subtract_88456/1 -> Product_88620/2
  Divide_4b770/1 -> Add_7e1c0/2

== system IEEE30_case/SG_D_23/d_E_fd_SG_D_23_block ==
  note: d_E_fd_SG_D_23 in IEEE30_case
      | $\frac{V_{f,\mathrm{SG},D,23}-E_{\mathrm{fd},\mathrm{SG},D,23}\,K_{E}}{T_{E}}$
      | Automatically generated on 2025-11-01 18:37:38 .
  State_E_fd_SG_D_23_30bc4 : Inport
  State_V_f_SG_D_23_7cc34 : Inport  Port=2
  Add_41652 : Sum
  Constant_-1_adc2a : Constant  Value=-1
  Constant_K_E_ff494 : Constant  Value=K_E
  Constant_T_E_21f5c : Constant  Value=T_E
  Divide_24900 : Product  Inputs=*/
  Product_a250d : Product
  Product_dc492 : Product
  Blockout_d_E_fd_SG_D_23_20bd2 : Outport
  wires:
  State_V_f_SG_D_23_7cc34/1 -> Add_41652/2
  Constant_-1_adc2a/1 -> Product_a250d/1
  State_E_fd_SG_D_23_30bc4/1 -> Product_a250d/2
  Constant_T_E_21f5c/1 -> Divide_24900/2
  Product_a250d/1 -> Product_dc492/1
  Constant_K_E_ff494/1 -> Product_dc492/2
  Add_41652/1 -> Divide_24900/1
  Divide_24900/1 -> Blockout_d_E_fd_SG_D_23_20bd2/1
  Product_dc492/1 -> Add_41652/1

== system IEEE30_case/SG_D_23/d_Px_1_SG_D_23_block ==
  note: d_Px_1_SG_D_23 in IEEE30_case
      | $\frac{w_{\mathrm{SG},D,23}-2\,\pi \,f_{0}}{T_{w}}-\frac{\mathrm{Px}_{1,\mathrm{SG},D,23}}{T_{w}}$
      | Automatically generated on 2025-11-01 18:37:39 .
  State_Px_1_SG_D_23_2554a : Inport
  State_w_SG_D_23_c0c14 : Inport  Port=2
  Add_2fda8 : Sum
  Add_feae4 : Sum
  Constant_-1_34014 : Constant  Value=-1
  Constant_-2.0_a63c5 : Constant  Value=-2.0
  Constant_T_w_48865 : Constant  Value=T_w
  Constant_T_w_de638 : Constant  Value=T_w
  Constant_f0_b9b83 : Constant  Value=f0
  Constant_pi_bd8cc : Constant  Value=pi
  Divide_878d8 : Product  Inputs=*/
  Divide_d9058 : Product  Inputs=*/
  Product_015be : Product
  Product_b1615 : Product
  Product_dcc41 : Product
  Blockout_d_Px_1_SG_D_23_e26cf : Outport
  wires:
  Constant_-2.0_a63c5/1 -> Product_dcc41/1
  Product_dcc41/1 -> Product_015be/1
  Product_015be/1 -> Add_2fda8/1
  Constant_pi_bd8cc/1 -> Product_dcc41/2
  Constant_f0_b9b83/1 -> Product_015be/2
  Constant_-1_34014/1 -> Product_b1615/1
  Divide_d9058/1 -> Add_feae4/1
  State_Px_1_SG_D_23_2554a/1 -> Product_b1615/2
  State_w_SG_D_23_c0c14/1 -> Add_2fda8/2
  Product_b1615/1 -> Divide_d9058/1
  Constant_T_w_48865/1 -> Divide_d9058/2
  Add_2fda8/1 -> Divide_878d8/1
  Constant_T_w_de638/1 -> Divide_878d8/2
  Divide_878d8/1 -> Add_feae4/2
  Add_feae4/1 -> Blockout_d_Px_1_SG_D_23_e26cf/1

== system IEEE30_case/SG_D_23/d_Px_2_SG_D_23_block ==
  note: d_Px_2_SG_D_23 in IEEE30_case
      | $\frac{\mathrm{Px}_{1,\mathrm{SG},D,23}-T_{2}\,\left(\frac{\mathrm{Px}_{1,\mathrm{SG},D,23}}{T_{w}}-\frac{w_{\mathrm{SG},D,23}-2\,\pi \,f_{0}}{T_{w}}\right)}{T_{1}}-\frac{\mathrm{Px}_{2,\mathrm{SG},D,23}}{T_{1}}$
      | Automatically generated on 2025-11-01 18:37:39 .
  State_Px_2_SG_D_23_3cd8e : Inport
  State_Px_1_SG_D_23_71728 : Inport  Port=2
  State_Px_1_SG_D_23_4e2ca : Inport  Port=3
  State_w_SG_D_23_f4d00 : Inport  Port=4
  Add_0a80b : Sum
  Add_0f3f5 : Sum
  Add_90232 : Sum
  Add_bca7c : Sum
  Constant_-1_0718f : Constant  Value=-1
  Constant_-1_4fc36 : Constant  Value=-1
  Constant_-2.0_32f52 : Constant  Value=-2.0
  Constant_T_1_31bc7 : Constant  Value=T_1
  Constant_T_1_da8ce : Constant  Value=T_1
  Constant_T_2_e50ab : Constant  Value=T_2
  Constant_T_w_0add9 : Constant  Value=T_w
  Constant_T_w_f7c58 : Constant  Value=T_w
  Constant_f0_522d8 : Constant  Value=f0
  Constant_pi_1ac13 : Constant  Value=pi
  Divide_70b6a : Product  Inputs=*/
  Divide_e2c8f : Product  Inputs=*/
  Divide_e7746 : Product  Inputs=*/
  Divide_f364a : Product  Inputs=*/
  Product_17a58 : Product
  Product_778e9 : Product
  Product_7a8ca : Product
  Product_9ccea : Product
  Product_aafa6 : Product
  Blockout_d_Px_2_SG_D_23_c0747 : Outport
  wires:
  Constant_-2.0_32f52/1 -> Product_17a58/1
  Product_17a58/1 -> Product_778e9/1
  Constant_pi_1ac13/1 -> Product_17a58/2
  State_Px_1_SG_D_23_4e2ca/1 -> Product_7a8ca/2
  Divide_f364a/1 -> Add_bca7c/1
  Constant_f0_522d8/1 -> Product_778e9/2
  Constant_-1_0718f/1 -> Product_7a8ca/1
  Constant_T_1_da8ce/1 -> Divide_f364a/2
  Product_778e9/1 -> Add_0f3f5/1
  State_w_SG_D_23_f4d00/1 -> Add_0f3f5/2
  Product_7a8ca/1 -> Divide_e2c8f/1
  Product_aafa6/1 -> Add_90232/2
  Constant_T_2_e50ab/1 -> Product_aafa6/1
  Constant_T_w_0add9/1 -> Divide_e2c8f/2
  Add_0f3f5/1 -> Divide_e7746/1
  Constant_T_w_f7c58/1 -> Divide_e7746/2
  Divide_e2c8f/1 -> Add_0a80b/1
  Divide_e7746/1 -> Add_0a80b/2
  Add_0a80b/1 -> Product_aafa6/2
  Constant_-1_4fc36/1 -> Product_9ccea/1
  State_Px_2_SG_D_23_3cd8e/1 -> Product_9ccea/2
  Add_90232/1 -> Divide_70b6a/1
  State_Px_1_SG_D_23_71728/1 -> Add_90232/1
  Product_9ccea/1 -> Divide_f364a/1
  Constant_T_1_31bc7/1 -> Divide_70b6a/2
  Divide_70b6a/1 -> Add_bca7c/2
  Add_bca7c/1 -> Blockout_d_Px_2_SG_D_23_c0747/1

== system IEEE30_case/SG_D_23/d_Px_3_SG_D_23_block ==
  note: d_Px_3_SG_D_23 in IEEE30_case
      | $\frac{\mathrm{Px}_{2,\mathrm{SG},D,23}+T_{4}\,\left(\frac{\mathrm{Px}_{1,\mathrm{SG},D,23}-T_{2}\,\left(\frac{\mathrm{Px}_{1,\mathrm{SG},D,23}}{T_{w}}-\frac{w_{\mathrm{SG},D,23}-2\,\pi \,f_{0}}{T_{w}}\right)}{T_{1}}-\frac{\mathrm{Px}_{2,\mathrm{SG},D,23}}{T_{1}}\right)}{T_{3}}-\frac{\mathrm{Px}_{3,\mathrm{SG},D,23}}{T_{3}}$
      | Automatically generated on 2025-11-01 18:37:42 .
  State_Px_3_SG_D_23_753eb : Inport
  State_Px_2_SG_D_23_11635 : Inport  Port=2
  State_Px_2_SG_D_23_48e63 : Inport  Port=3
  State_Px_1_SG_D_23_327f4 : Inport  Port=4
  State_Px_1_SG_D_23_5f089 : Inport  Port=5
  State_w_SG_D_23_9958b : Inport  Port=6
  Add_18ef5 : Sum
  Add_376d8 : Sum
  Add_7abe7 : Sum
  Add_ca90d : Sum
  Add_da040 : Sum
  Add_ed61e : Sum
  Constant_-1_40fc2 : Constant  Value=-1
  Constant_-1_9a309 : Constant  Value=-1
  Constant_-1_d1f4d : Constant  Value=-1
  Constant_-2.0_b17de : Constant  Value=-2.0
  Constant_T_1_26354 : Constant  Value=T_1
  Constant_T_1_68678 : Constant  Value=T_1
  Constant_T_2_0b479 : Constant  Value=T_2
  Constant_T_3_00049 : Constant  Value=T_3
  Constant_T_3_e4b69 : Constant  Value=T_3
  Constant_T_4_1e132 : Constant  Value=T_4
  Constant_T_w_1733e : Constant  Value=T_w
  Constant_T_w_82a78 : Constant  Value=T_w
  Constant_f0_2d4d6 : Constant  Value=f0
  Constant_pi_e0132 : Constant  Value=pi
  Divide_223c5 : Product  Inputs=*/
  Divide_3562e : Product  Inputs=*/
  Divide_42ad1 : Product  Inputs=*/
  Divide_47f51 : Product  Inputs=*/
  Divide_8051b : Product  Inputs=*/
  Divide_b28b0 : Product  Inputs=*/
  Product_371bc : Product
  Product_722ee : Product
  Product_725c0 : Product
  Product_8152b : Product
  Product_96e25 : Product
  Product_dd44a : Product
  Product_ee2ce : Product
  Blockout_d_Px_3_SG_D_23_d0055 : Outport
  wires:
  Constant_-2.0_b17de/1 -> Product_ee2ce/1
  Constant_pi_e0132/1 -> Product_ee2ce/2
  Product_ee2ce/1 -> Product_8152b/1
  State_Px_1_SG_D_23_5f089/1 -> Product_dd44a/2
  Divide_b28b0/1 -> Add_376d8/2
  Constant_f0_2d4d6/1 -> Product_8152b/2
  Constant_T_3_e4b69/1 -> Divide_47f51/2
  Constant_-1_40fc2/1 -> Product_dd44a/1
  Product_8152b/1 -> Add_da040/1
  Add_da040/1 -> Divide_b28b0/1
  State_w_SG_D_23_9958b/1 -> Add_da040/2
  Constant_T_1_26354/1 -> Divide_42ad1/2
  Product_dd44a/1 -> Divide_3562e/1
  Constant_T_w_1733e/1 -> Divide_3562e/2
  Constant_T_w_82a78/1 -> Divide_b28b0/2
  Divide_3562e/1 -> Add_376d8/1
  Constant_T_3_00049/1 -> Divide_8051b/2
  Product_96e25/1 -> Add_ca90d/2
  Constant_T_2_0b479/1 -> Product_96e25/1
  Add_376d8/1 -> Product_96e25/2
  Constant_T_1_68678/1 -> Divide_223c5/2
  Product_371bc/1 -> Divide_223c5/1
  Constant_-1_d1f4d/1 -> Product_371bc/1
  State_Px_2_SG_D_23_48e63/1 -> Product_371bc/2
  Add_7abe7/1 -> Blockout_d_Px_3_SG_D_23_d0055/1
  Add_ca90d/1 -> Divide_42ad1/1
  State_Px_1_SG_D_23_327f4/1 -> Add_ca90d/1
  Divide_223c5/1 -> Add_ed61e/1
  Divide_42ad1/1 -> Add_ed61e/2
  Product_722ee/1 -> Add_18ef5/2
  Constant_T_4_1e132/1 -> Product_722ee/1
  Add_ed61e/1 -> Product_722ee/2
  Constant_-1_9a309/1 -> Product_725c0/1
  State_Px_3_SG_D_23_753eb/1 -> Product_725c0/2
  Divide_8051b/1 -> Add_7abe7/1
  Add_18ef5/1 -> Divide_47f51/1
  State_Px_2_SG_D_23_11635/1 -> Add_18ef5/1
  Product_725c0/1 -> Divide_8051b/1
  Divide_47f51/1 -> Add_7abe7/2

== system IEEE30_case/SG_D_23/d_R_f_SG_D_23_block ==
  note: d_R_f_SG_D_23 in IEEE30_case
      | $-\frac{R_{f,\mathrm{SG},D,23}-\frac{E_{\mathrm{fd},\mathrm{SG},D,23}\,K_{F}}{T_{F}}}{T_{F}}$
      | Automatically generated on 2025-11-01 18:37:38 .
  State_E_fd_SG_D_23_12145 : Inport
  State_R_f_SG_D_23_3a056 : Inport  Port=2
  Constant_K_F_856b7 : Constant  Value=K_F
  Constant_T_F_4dd45 : Constant  Value=T_F
  Constant_T_F_c2850 : Constant  Value=T_F
  Divide_011af : Product  Inputs=*/
  Divide_b674a : Product  Inputs=*/
  Product_65e86 : Product
  Subtract_8b298 : Sum  Inputs=+-
  Blockout_d_R_f_SG_D_23_d5fff : Outport
  wires:
  State_E_fd_SG_D_23_12145/1 -> Product_65e86/1
  Constant_K_F_856b7/1 -> Product_65e86/2
  Product_65e86/1 -> Divide_b674a/1
  Divide_b674a/1 -> Subtract_8b298/1
  Constant_T_F_c2850/1 -> Divide_b674a/2
  State_R_f_SG_D_23_3a056/1 -> Subtract_8b298/2
  Constant_T_F_4dd45/1 -> Divide_011af/2
  Subtract_8b298/1 -> Divide_011af/1
  Divide_011af/1 -> Blockout_d_R_f_SG_D_23_d5fff/1

== system IEEE30_case/SG_D_23/d_T_m_SG_D_23_block ==
  note: d_T_m_SG_D_23 in IEEE30_case
      | $-\frac{T_{m,\mathrm{SG},D,23}-T_{0}+\frac{\mathrm{SpeedPara}\,\left(w_{\mathrm{SG},D,23}-w_{\mathrm{ref}}\right)}{2\,f_{0}\,\pi }}{T_{\mathrm{speed}}}$
      | Automatically generated on 2025-11-01 18:37:29 .
  State_w_SG_D_23_66b81 : Inport
  State_T_m_SG_D_23_81d1e : Inport  Port=2
  Add_28797 : Sum
  Add_b6d58 : Sum
  Constant_-1_d5486 : Constant  Value=-1
  Constant_2.0_88d3f : Constant  Value=2.0
  Constant_SpeedPara_f9be5 : Constant  Value=SpeedPara
  Constant_T_0_8b36a : Constant  Value=T_0
  Constant_T_speed_1c562 : Constant  Value=T_speed
  Constant_f0_d4846 : Constant  Value=f0
  Constant_pi_ee4f4 : Constant  Value=pi
  Constant_w_ref_d7e69 : Constant  Value=w_ref
  Divide_21e78 : Product  Inputs=*/
  Divide_620bb : Product  Inputs=*/
  Product_0ce1b : Product
  Product_2b2be : Product
  Product_7fc53 : Product
  Product_a9589 : Product
  Subtract_e2bb9 : Sum  Inputs=+-
  Blockout_d_T_m_SG_D_23_c269a : Outport
  wires:
  State_w_SG_D_23_66b81/1 -> Product_7fc53/2
  Constant_SpeedPara_f9be5/1 -> Product_a9589/1
  Constant_-1_d5486/1 -> Product_7fc53/1
  Constant_2.0_88d3f/1 -> Product_2b2be/1
  Product_7fc53/1 -> Add_28797/1
  Constant_w_ref_d7e69/1 -> Add_28797/2
  Add_28797/1 -> Product_a9589/2
  Constant_pi_ee4f4/1 -> Product_2b2be/2
  Product_2b2be/1 -> Product_0ce1b/1
  Constant_f0_d4846/1 -> Product_0ce1b/2
  Product_a9589/1 -> Divide_21e78/1
  Product_0ce1b/1 -> Divide_21e78/2
  Divide_21e78/1 -> Add_b6d58/1
  Constant_T_0_8b36a/1 -> Add_b6d58/2
  Add_b6d58/1 -> Subtract_e2bb9/1
  State_T_m_SG_D_23_81d1e/1 -> Subtract_e2bb9/2
  Subtract_e2bb9/1 -> Divide_620bb/1
  Constant_T_speed_1c562/1 -> Divide_620bb/2
  Divide_620bb/1 -> Blockout_d_T_m_SG_D_23_c269a/1
